simulink model "DigitalPIDWithFilter"  (R2021a)
settings: Solver=VariableStepAuto  StartTime=0.0  StopTime=SimTime-Ts  RelTol=1e-3
values from neighbouring files (symbols this model uses):
  C12 = x(3)    [DigitalPIDRunner.m]    (also in DoubleMassRunner.m; NNIdentify.m = Xnt_noise(3); NNTrainingSet.m = T(i, 3); PIDModalController.m = 16.6338)
  d_prz0 = Ki*Tq^2 - 2*Kp*Tq + 4*Kd    (= 3.99401)    [DigitalPIDRunner.m]
  d_prz1 = 2*Ki*Tq^2 - 8*Kd    (= -7.99998)    [DigitalPIDRunner.m]
  d_prz2 = Ki*Tq^2 + 2*Kp*Tq + 4*Kd    (= 4.00601)    [DigitalPIDRunner.m]
  dz0 = 2*Tq    (= 0.002)    [DigitalPIDRunner.m]
  dz1 = -8*Tq    (= -0.008)    [DigitalPIDRunner.m]
  dz2 = 6*Tq    (= 0.006)    [DigitalPIDRunner.m]
  k1 = x(1)    [DigitalPIDRunner.m]    (also in DoubleMassRunner.m; NNIdentify.m = Xnt_noise(1); NNTrainingSet.m = T(i, 1); PIDModalController.m = 0.2244)
  k2 = x(2)    [DigitalPIDRunner.m]    (also in DoubleMassRunner.m; NNIdentify.m = Xnt_noise(2); NNTrainingSet.m = T(i, 2); PIDModalController.m = 0.5636)
  Kd = 1    [DigitalPIDRunner.m]    (also in PIDModalController.m = (a2j*Omega - a1)/b0; PIDRunner.m = X(3); PolynomialController.m = (a2j*Omega - a1)/b0)
  Ki = 10    [DigitalPIDRunner.m]    (also in PIDModalController.m = (a0j*Omega^3)/b0; PIDRunner.m = X(2); PolynomialController.m = (a0j*Omega^3)/b0)
  Kp = 3    [DigitalPIDRunner.m]    (also in PIDModalController.m = (a1j*Omega^2 - a0)/b0; PIDRunner.m = X(1); PolynomialController.m = (a1j*Omega^2 - a0)/b0)
  n_prz0 = Ki*Tq^2    (= 1e-05)    [DigitalPIDRunner.m]
  n_prz1 = 2*Ki*Tq^2    (= 2e-05)    [DigitalPIDRunner.m]
  n_prz2 = Ki*Tq^2    (= 1e-05)    [DigitalPIDRunner.m]
  nz0 = Ki*Tq^2 - 2*Kp*Tq + 4*Kd    (= 3.99401)    [DigitalPIDRunner.m]
  nz1 = (2*Ki*Tq^2 - 8*Kd)    (= -7.99998)    [DigitalPIDRunner.m]
  nz2 = (Ki*Tq^2 + 2*Kp*Tq + 4*Kd)    (= 4.00601)    [DigitalPIDRunner.m]
  Tq = 1e-2    (= 0.01)    [ComparisonDiscresization.m]    (also in DigitalPIDRunner.m = 0.001; NNTrainingSet.m = 0.1; reference.mat = 0.1)
  Ts = 1e-3    (= 0.001)    [DigitalPIDRunner.m]    (also in DoubleMassRunner.m = ref.Ts; NNTrainingSet.m; PIDModalController.m; PIDRunner.m = p.Results.StepTime)
settings Model: Creator=akangmufti  LastModifiedBy=akangmufti

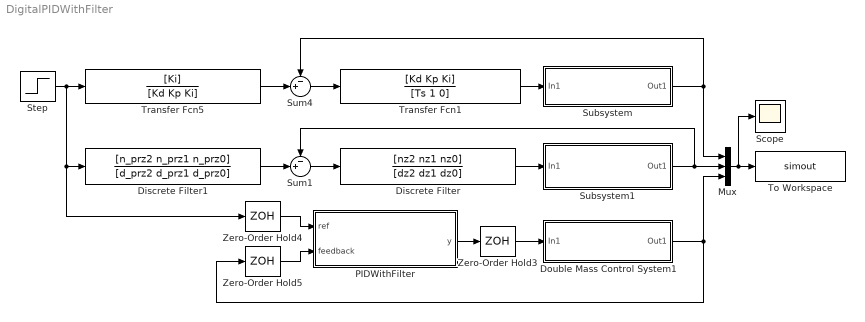
== system DigitalPIDWithFilter ==
  Discrete Filter : DiscreteFilter  Numerator=[nz2 nz1 nz0]  Denominator=[dz2 dz1 dz0]  SampleTime=Ts
  Discrete Filter1 : DiscreteFilter  Numerator=[n_prz2 n_prz1 n_prz0]  Denominator=[d_prz2 d_prz1 d_prz0]  SampleTime=Ts
  Double Mass Control System1 : Subsystem
  Mux : Mux  Inputs=3
  PIDWithFilter : MATLAB Function  TreatAsAtomicUnit=on
  Scope : Scope
  Step : Step  Time=Tq  SampleTime=0
  Subsystem : Subsystem
  Subsystem1 : Subsystem
  Sum1 : Sum  Inputs=-+|
  Sum4 : Sum  Inputs=-+|
  To Workspace : ToWorkspace  VariableName=simout  SampleTime=-1
      settings: Save2DSignal=2-D array (concatenate along first dimension)
  Transfer Fcn1 : TransferFcn  Numerator=[Kd Kp Ki]  Denominator=[Ts 1 0]
  Transfer Fcn5 : TransferFcn  Numerator=[Ki]  Denominator=[Kd Kp Ki]
  Zero-Order Hold3 : ZeroOrderHold  SampleTime=Ts
  Zero-Order Hold4 : ZeroOrderHold  SampleTime=Ts
  Zero-Order Hold5 : ZeroOrderHold  SampleTime=Ts
  wires:
  Zero-Order Hold4/1 -> PIDWithFilter/1(ref)
  Zero-Order Hold5/1 -> PIDWithFilter/2(feedback)
  Step/1 -> Zero-Order Hold4/1, Discrete Filter1/1, Transfer Fcn5/1
  Double Mass Control System1/1(Out1) -> Mux/3, Zero-Order Hold5/1
  Zero-Order Hold3/1 -> Double Mass Control System1/1(In1)
  PIDWithFilter/1(y) -> Zero-Order Hold3/1
  Transfer Fcn1/1 -> Subsystem/1(In1)
  Subsystem/1(Out1) -> Sum4/1, Mux/1
  Transfer Fcn5/1 -> Sum4/2
  Sum4/1 -> Transfer Fcn1/1
  Mux/1 -> Scope/1, To Workspace/1
  Discrete Filter/1 -> Subsystem1/1(In1)
  Sum1/1 -> Discrete Filter/1
  Discrete Filter1/1 -> Sum1/2
  Subsystem1/1(Out1) -> Sum1/1, Mux/2

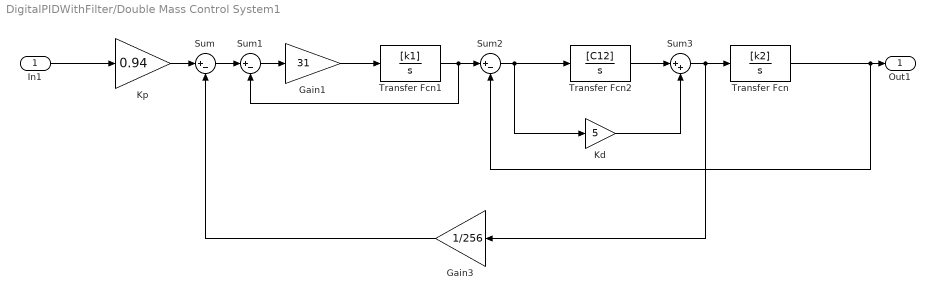
== system DigitalPIDWithFilter/Double Mass Control System1 ==
  In1 : Inport
  Gain1 : Gain  Gain=31
  Gain3 : Gain  Gain=1/256
  Kd : Gain  Gain=5
  Kp : Gain  Gain=0.94
  Sum : Sum  Inputs=|+-
  Sum1 : Sum  Inputs=|+-
  Sum2 : Sum  Inputs=|+-
  Sum3 : Sum  Inputs=|++
  Transfer Fcn : TransferFcn  Numerator=[k2]  Denominator=[1 0]
  Transfer Fcn1 : TransferFcn  Numerator=[k1]  Denominator=[1 0]
  Transfer Fcn2 : TransferFcn  Numerator=[C12]  Denominator=[1 0]
  Out1 : Outport
  wires:
  Kp/1 -> Sum/1
  Transfer Fcn1/1 -> Sum2/1, Sum1/2
  Gain1/1 -> Transfer Fcn1/1
  Sum2/1 -> Kd/1, Transfer Fcn2/1
  Sum1/1 -> Gain1/1
  Gain3/1 -> Sum/2
  Sum/1 -> Sum1/1
  Sum3/1 -> Transfer Fcn/1, Gain3/1
  Transfer Fcn2/1 -> Sum3/1
  In1/1 -> Kp/1
  Kd/1 -> Sum3/2
  Transfer Fcn/1 -> Sum2/2, Out1/1

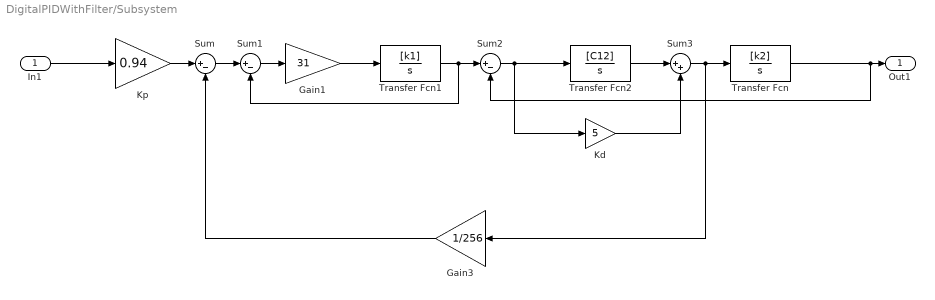
== system DigitalPIDWithFilter/Subsystem ==
  In1 : Inport
  Gain1 : Gain  Gain=31
  Gain3 : Gain  Gain=1/256
  Kd : Gain  Gain=5
  Kp : Gain  Gain=0.94
  Sum : Sum  Inputs=|+-
  Sum1 : Sum  Inputs=|+-
  Sum2 : Sum  Inputs=|+-
  Sum3 : Sum  Inputs=|++
  Transfer Fcn : TransferFcn  Numerator=[k2]  Denominator=[1 0]
  Transfer Fcn1 : TransferFcn  Numerator=[k1]  Denominator=[1 0]
  Transfer Fcn2 : TransferFcn  Numerator=[C12]  Denominator=[1 0]
  Out1 : Outport
  wires:
  Kp/1 -> Sum/1
  Transfer Fcn1/1 -> Sum2/1, Sum1/2
  Gain1/1 -> Transfer Fcn1/1
  Sum2/1 -> Kd/1, Transfer Fcn2/1
  Sum1/1 -> Gain1/1
  Gain3/1 -> Sum/2
  Sum/1 -> Sum1/1
  Sum3/1 -> Transfer Fcn/1, Gain3/1
  Transfer Fcn2/1 -> Sum3/1
  In1/1 -> Kp/1
  Kd/1 -> Sum3/2
  Transfer Fcn/1 -> Sum2/2, Out1/1

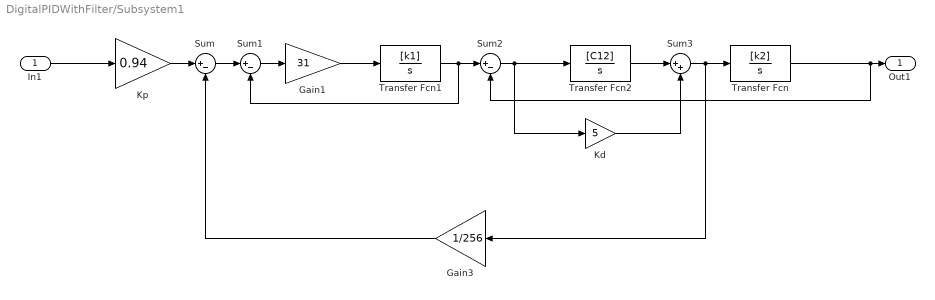
== system DigitalPIDWithFilter/Subsystem1 ==
  In1 : Inport
  Gain1 : Gain  Gain=31
  Gain3 : Gain  Gain=1/256
  Kd : Gain  Gain=5
  Kp : Gain  Gain=0.94
  Sum : Sum  Inputs=|+-
  Sum1 : Sum  Inputs=|+-
  Sum2 : Sum  Inputs=|+-
  Sum3 : Sum  Inputs=|++
  Transfer Fcn : TransferFcn  Numerator=[k2]  Denominator=[1 0]
  Transfer Fcn1 : TransferFcn  Numerator=[k1]  Denominator=[1 0]
  Transfer Fcn2 : TransferFcn  Numerator=[C12]  Denominator=[1 0]
  Out1 : Outport
  wires:
  Kp/1 -> Sum/1
  Transfer Fcn1/1 -> Sum2/1, Sum1/2
  Gain1/1 -> Transfer Fcn1/1
  Sum2/1 -> Kd/1, Transfer Fcn2/1
  Sum1/1 -> Gain1/1
  Gain3/1 -> Sum/2
  Sum/1 -> Sum1/1
  Sum3/1 -> Transfer Fcn/1, Gain3/1
  Transfer Fcn2/1 -> Sum3/1
  In1/1 -> Kp/1
  Kd/1 -> Sum3/2
  Transfer Fcn/1 -> Sum2/2, Out1/1

== matlab function DigitalPIDWithFilter/PIDWithFilter ==
  data: ref input; feedback input; y output
function y = PIDWithFilter(ref, feedback)
    persistent yk yk_1 yk_2 xk xk_1 xk_2
    persistent ykf yk_1f yk_2f xkf xk_1f xk_2f
    if(isempty(yk))
        yk     = 0;
        yk_1   = 0;
        yk_2   = 0;
        xk     = 0;
        xk_1   = 0;
        xk_2   = 0;
        
        ykf     = 0;
        yk_1f   = 0;
        yk_2f   = 0;
        xkf     = 0;
        xk_1f   = 0;
        xk_2f   = 0;
    end

    % Coefficients for continous time PID controler
    Kp = 33.4244;
    Ki = 114.9607;
    Kd = 3.1197;
    Tq   = 0.001;

nz2 = (Ki*Tq^2 + 2*Kp*Tq + 4*Kd);
nz1 = (2*Ki*Tq^2 - 8*Kd);
nz0 = Ki*Tq^2 - 2*Kp*Tq + 4*Kd;

dz2 = 6*Tq;
dz1 = -8*Tq;
dz0 = 2*Tq;

n_prz0 = Ki*Tq^2;
n_prz1 = 2*Ki*Tq^2;
n_prz2 = Ki*Tq^2;

d_prz0 = Ki*Tq^2 - 2*Kp*Tq + 4*Kd;
d_prz1 = 2*Ki*Tq^2 - 8*Kd;
d_prz2 = Ki*Tq^2 + 2*Kp*Tq + 4*Kd;

xkf = ref;
ykf = (xkf*n_prz2 + xk_1f*n_prz1 + xk_2f*n_prz0 - (yk_1f*d_prz1 + yk_2f*d_prz0)) / d_prz2;
yk_2f = yk_1f;
yk_1f = ykf;    
xk_2f = xk_1f;
xk_1f = xkf;

xk = ykf - feedback;
yk = (xk*nz2 + xk_1*nz1 + xk_2*nz0 - (yk_1*dz1 + yk_2*dz0)) / dz2;
yk_2 = yk_1;
yk_1 = yk;    
xk_2 = xk_1;
xk_1 = xk;

y = yk;
